simulink model "Receive1"  (R2021a)
settings: Solver=VariableStepAuto  StartTime=0.0  StopTime=20000  RelTol=1e-3
values from neighbouring files (symbols this model uses):
  n_overlapped_channel = 2 * 1024    (= 2048)    [receive1_script.m]
  parallel_factor = 4    [receive1_script.m]
libraries: xbsIndex_r4 x522, xrbsSSR_Library x15, dspsrcs4 x12
(part 1 of 4)
settings Model: Creator=11037  LastModifiedBy=11037

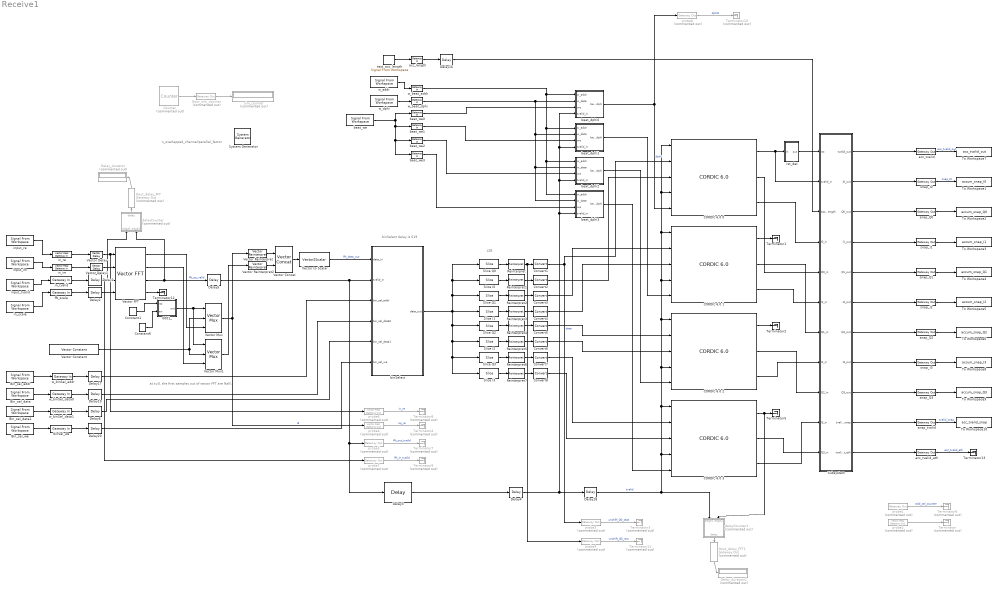
== system Receive1 ==
  note: binSelect delay is 519
  note: n_overlapped_channel/parallel_factor
  note: LSB
  note: at t=0, the first samples out of vector FFT are NaN,
  " System Generator" : xbsIndex_r4/ System Generator  Tag=genX  xilinxfamily=zynquplusRFSOC  part=xczu28dr  speed=-2-e  package=ffvg1517  synthesis_tool=Vivado  clock_wrapper=Clock Enables  directory=C:/Receive1_test_NL  proj_type=Vivado  Synth_file=Vivado Synthesis Defaults  Impl_file=Vivado Implementation Defaults  testbench=off  simulink_period=1  sysclk_period=10  dcm_input_clock_period=10  incr_netlist=off  trim_vbits=Everywhere in SubSystem  dbl_ovrd=According to Block Masks  core_generation=According to Block Masks  run_coregen=off  deprecated_control=off  eval_field=0  block_type=sysgen
  0001_ : Subsystem
  Bin_sel_addr : dspsrcs4/Signal From Workspace  X=15  Ts=1  nsamps=1  OutputAfterFinalValue=Holding final value  ignoreOrWarnInputAndFrameLengths=on  OutputFrames=off
  Bin_sel_data : dspsrcs4/Signal From Workspace  X=15  Ts=1  nsamps=1  OutputAfterFinalValue=Holding final value  ignoreOrWarnInputAndFrameLengths=on  OutputFrames=off
  Bin_sel_data1 : dspsrcs4/Signal From Workspace  X=15  Ts=1  nsamps=1  OutputAfterFinalValue=Holding final value  ignoreOrWarnInputAndFrameLengths=on  OutputFrames=off
  Bin_sel_we : dspsrcs4/Signal From Workspace  X=0  Ts=1  nsamps=1  OutputAfterFinalValue=Setting to zero  ignoreOrWarnInputAndFrameLengths=on  OutputFrames=off
  CORDIC 6.0 {0..3} (4 alike) : xbsIndex_r4/CORDIC 6.0   functional_selection=Rotate  architectural_configuration=Parallel  pipelining_mode=Optimal  data_format=SignedFraction  phase_format=Scaled_Radians  input_width=18  output_width=16  round_mode=Nearest_Even  iterations=16  precision=20  compensation_scaling=LUT_based  coarse_rotation=on  aclken=off  aresetn=off  out_tready=off  cartesian_has_tuser=off  cartesian_has_tlast=off  cartesian_tuser_width=1  phase_has_tuser=off  phase_has_tlast=off  phase_tuser_width=1  out_tlast_behv=Null  flow_control=NonBlocking  optimize_goal=Resources  trim_axipin_name=on  simulation_type=hybrid_sim  simulation_model=sysgen:cordic_v6_0  data_path_portlist={'s_axis_cartesian_tdata_imag', 's_axis_cartesian_tdata_real', 's_axis_phase_tdata_phase', 'm_axis_dout_tdata_imag', 'm_axis_dout_tdata_real', 'm_axis_dout_tdata_phase','m_axis_dout_tdata'}  ip_name=CORDIC  ip_version=6.0  dsptool_ready=true  ipcore_usecache=true  ipcore_useipmodelcache=true  wrapper_available=true  port_translation_map={ 'aclken' => 'en', 'aresetn' => 'rst' }  block_type=cordic_v6_0
      settings: infoedit=CORDIC 6.0
  Constant1 : xbsIndex_r4/Constant  const=0  gui_display_data_type=Boolean  arith_type=Boolean  n_bits=16  bin_pt=14  preci_type=Single  exp_width=8  frac_width=24  explicit_period=on  period=1  equ=P=C  opselect=C  inp2=PCIN>>17  opr=+  inp1=P  carry=CIN  dbl_ovrd=off  block_type=constant
  Constant6 : xbsIndex_r4/Constant  const=1  gui_display_data_type=Boolean  arith_type=Boolean  n_bits=16  bin_pt=14  preci_type=Single  exp_width=8  frac_width=24  explicit_period=on  period=1  equ=P=C  opselect=C  inp2=PCIN>>17  opr=+  inp1=P  carry=CIN  dbl_ovrd=off  block_type=constant
  Convert{1..8} (8 alike) : xbsIndex_r4/Convert  gui_display_data_type=Fixed-point  arith_type="Signed  (2's comp)"  n_bits=18  bin_pt=16  float_type=Single  exp_bits=8  fraction_bits=24  quantization=Truncate  overflow=Flag as error  en=off  latency=1  pipeline=off  dbl_ovrd=off  block_type=convert
  Counter : xbsIndex_r4/Counter  Commented=on  cnt_type=Free Running  cnt_to=Inf  operation=Up  start_count=0  cnt_by_val=1  arith_type=Unsigned  n_bits=24  bin_pt=0  load_pin=off  rst=off  en=off  explicit_period=on  period=1  use_behavioral_HDL=off  implementation=Fabric  dbl_ovrd=off  block_type=counter
  Delay1 : xbsIndex_r4/Delay  rst=off  infoeditControl=Selection of Reset will increase slice count due to use of real FFs and instead of SRLs  en=off  latency=1+15*256  reg_retiming=off  dbl_ovrd=off  block_type=delay
  Delay{2,4..6,16..17,19..20} (8 alike) : xbsIndex_r4/Delay  rst=off  infoeditControl=Selection of Reset will increase slice count due to use of real FFs and instead of SRLs  en=off  latency=1  reg_retiming=off  dbl_ovrd=off  block_type=delay
  Delay18 : xbsIndex_r4/Delay  rst=off  infoeditControl=Selection of Reset will increase slice count due to use of real FFs and instead of SRLs  en=off  latency=2  reg_retiming=off  dbl_ovrd=off  block_type=delay
  Delay3 : xbsIndex_r4/Delay  rst=off  infoeditControl=Selection of Reset will increase slice count due to use of real FFs and instead of SRLs  en=off  latency=519-2  reg_retiming=off  dbl_ovrd=off  block_type=delay
  Delay_duration : Display  Commented=on
  Delay_duration1 : Display  Commented=on
  Gout_delay_FFT : xbsIndex_r4/Gateway Out  Commented=on  inherit_from_input=on  hdl_port=on  rows=1  columns=1  UseAsDAC=off  DACChannel='1'  interface=None  automatic_assignment=on  address_offset=hex2dec('00')  intf_name=''  intf_description=''  timing_constraint=None  locs_specified=off  LOCs={}  io_standard={}  block_type=gatewayout
  Gout_delay_FFT1 : xbsIndex_r4/Gateway Out  Commented=on  inherit_from_input=on  hdl_port=on  rows=1  columns=1  UseAsDAC=off  DACChannel='1'  interface=None  automatic_assignment=on  address_offset=hex2dec('00')  intf_name=''  intf_description=''  timing_constraint=None  locs_specified=off  LOCs={}  io_standard={}  block_type=gatewayout
  Gout_sim_counter : xbsIndex_r4/Gateway Out  Commented=on  inherit_from_input=on  hdl_port=on  rows=1  columns=1  UseAsDAC=off  DACChannel='1'  interface=None  automatic_assignment=on  address_offset=hex2dec('00')  intf_name=''  intf_description=''  timing_constraint=None  locs_specified=off  LOCs={}  io_standard={}  block_type=gatewayout
  Reinterpret{,1..7} (8 alike) : xbsIndex_r4/Reinterpret  force_arith_type=on  arith_type="Signed  (2's comp)"  force_bin_pt=on  bin_pt=15  block_type=reinterpret
  Slice I0 : xbsIndex_r4/Slice  nbits=27  boolean_output=off  mode=Lower Bit Location + Width  bit1=0  base1=MSB of Input  bit0=27  base0=LSB of Input  dbl_ovrd=off  block_type=slice
  Slice I1 : xbsIndex_r4/Slice  nbits=27  boolean_output=off  mode=Lower Bit Location + Width  bit1=0  base1=MSB of Input  bit0=27*3  base0=LSB of Input  dbl_ovrd=off  block_type=slice
  Slice I2 : xbsIndex_r4/Slice  nbits=27  boolean_output=off  mode=Lower Bit Location + Width  bit1=0  base1=MSB of Input  bit0=27*5  base0=LSB of Input  dbl_ovrd=off  block_type=slice
  Slice I3 : xbsIndex_r4/Slice  nbits=27  boolean_output=off  mode=Lower Bit Location + Width  bit1=0  base1=MSB of Input  bit0=27*7  base0=LSB of Input  dbl_ovrd=off  block_type=slice
  Slice Q0 : xbsIndex_r4/Slice  nbits=27  boolean_output=off  mode=Lower Bit Location + Width  bit1=0  base1=MSB of Input  bit0=0  base0=LSB of Input  dbl_ovrd=off  block_type=slice
  Slice Q1 : xbsIndex_r4/Slice  nbits=27  boolean_output=off  mode=Lower Bit Location + Width  bit1=0  base1=MSB of Input  bit0=27*2  base0=LSB of Input  dbl_ovrd=off  block_type=slice
  Slice Q2 : xbsIndex_r4/Slice  nbits=27  boolean_output=off  mode=Lower Bit Location + Width  bit1=0  base1=MSB of Input  bit0=27*4  base0=LSB of Input  dbl_ovrd=off  block_type=slice
  Slice Q3 : xbsIndex_r4/Slice  nbits=27  boolean_output=off  mode=Lower Bit Location + Width  bit1=0  base1=MSB of Input  bit0=27*6  base0=LSB of Input  dbl_ovrd=off  block_type=slice
  Subsystem : Subsystem
  Terminator{,3..4,6..11} (9 alike) : Terminator  Commented=on
  Terminator{1..2,5,12..13} (5 alike) : Terminator
  To Workspace1 : ToWorkspace  VariableName=accum_snap_I0  SampleTime=1
  To Workspace10 : ToWorkspace  VariableName=acc_tvalid_snap  SampleTime=1
  To Workspace2 : ToWorkspace  VariableName=accum_snap_Q0  SampleTime=1
  To Workspace3 : ToWorkspace  VariableName=accum_snap_I1  SampleTime=1
  To Workspace4 : ToWorkspace  VariableName=accum_snap_Q1  SampleTime=1
  To Workspace5 : ToWorkspace  VariableName=accum_snap_I2  SampleTime=1
  To Workspace6 : ToWorkspace  VariableName=accum_snap_Q2  SampleTime=1
  To Workspace7 : ToWorkspace  VariableName=acc_tvalid_out  SampleTime=1
  To Workspace8 : ToWorkspace  VariableName=accum_snap_I3  SampleTime=1
  To Workspace9 : ToWorkspace  VariableName=accum_snap_Q3  SampleTime=1
  Vector Concat : xrbsSSR_Library/Vector Concat  num_inputs=2  num_inputs_prev=2  sg_ssr=4  sg_ssr_prev=4  dbl_ovrd=off  block_type=concat_ssr  sg_ssr_name=vect_concat
      settings: SourceProductName=Xilinx SSR Blockset  infoedit=The Vector Concat block concatenates two or more inputs of type vector. Output will be cast to an unsigned value with the binary point at zero.
  Vector Constant : xrbsSSR_Library/Vector Constant  const=[0.9 0.9 0.9 0.9]  gui_display_data_type=Fixed-point  arith_type=Signed (2's comp)  n_bits=16  bin_pt=15  preci_type=Single  exp_width=8  frac_width=24  explicit_period=on  period=1  sg_ssr=4  sg_ssr_prev=4  equ=P=C  opselect=C  inp2=PCIN>>17  opr=+  inp1=P  carry=CIN  dbl_ovrd=off  block_type=constant_ssr
      settings: SourceProductName=Xilinx SSR Blockset
  Vector Delay : xrbsSSR_Library/Vector Delay  sg_latency=1  infoeditControl=Selection of Reset will increase slice count due to use of real FFs and instead of SRLs  en=off  vectorize_en=off  rst=off  reg_retiming=off  block_type=delay_ssr  dbl_ovrd=off  sg_ssr=4  sg_ssr_prev=4  sg_ssr_name=vect_delay
      settings: SourceProductName=Xilinx SSR Blockset
  Vector Delay1 : xrbsSSR_Library/Vector Delay  sg_latency=1  infoeditControl=Selection of Reset will increase slice count due to use of real FFs and instead of SRLs  en=off  vectorize_en=off  rst=off  reg_retiming=off  block_type=delay_ssr  dbl_ovrd=off  sg_ssr=4  sg_ssr_prev=4  sg_ssr_name=vect_delay
      settings: SourceProductName=Xilinx SSR Blockset
  Vector FFT : xrbsSSR_Library/Vector FFT  sg_ssr=4  N=2048  W_high=1  W_low=-17  n_bits=27  bin_pt=14+1  bram_threshold=258  block_type=fft_ssr  sg_ssr_prev=4
      settings: SourceProductName=Xilinx SSR Blockset
  Vector Mux : xrbsSSR_Library/Vector Mux  inputs=2  inputs_prev=2  en=off  vectorize_en=off  vectorize_sel=off  sg_latency=1  precision=User Defined  arith_type="Signed  (2's comp)"  n_bits=27  bin_pt=15  quantization=Truncate  overflow=Saturate  dbl_ovrd=off  block_type=mux_ssr  sg_ssr=4  sg_ssr_prev=4  sg_ssr_name=vect_mux
      settings: SourceProductName=Xilinx SSR Blockset  infoedit=The Vector Multiplexer block supports Multiplexing feature for input of vector types.
  Vector Mux1 : xrbsSSR_Library/Vector Mux  inputs=2  inputs_prev=2  en=off  vectorize_en=off  vectorize_sel=off  sg_latency=1  precision=User Defined  arith_type="Signed  (2's comp)"  n_bits=27  bin_pt=15  quantization=Truncate  overflow=Saturate  dbl_ovrd=off  block_type=mux_ssr  sg_ssr=4  sg_ssr_prev=4  sg_ssr_name=vect_mux
      settings: SourceProductName=Xilinx SSR Blockset  infoedit=The Vector Multiplexer block supports Multiplexing feature for input of vector types.
  Vector Reinterpret : xrbsSSR_Library/Vector Reinterpret  sg_ssr=4  sg_ssr_prev=4  force_arith_type=on  arith_type=Unsigned  force_bin_pt=on  bin_pt=0  block_type=reinterpret_ssr
      settings: SourceProductName=Xilinx SSR Blockset  infoedit="The Vector Reinterpret block Changes vector input signal type without altering the binary representation. You can change the signal between signed and unsigned, and relocate the binary point.<br><br>Hardware notes: In hardware this block costs nothing.<br><br>Example:  Suppose the input is 6 bits wide, signed, with 2 fractional bits, and the output is forced to unsigned with 0 fractional bits.  Then an input of -2.0 (1110.00 in binary 2's complement) becomes an output of 56 (111000 in binary)."
  Vector Reinterpret2 : xrbsSSR_Library/Vector Reinterpret  sg_ssr=4  sg_ssr_prev=4  force_arith_type=on  arith_type=Unsigned  force_bin_pt=on  bin_pt=0  block_type=reinterpret_ssr
      settings: SourceProductName=Xilinx SSR Blockset  infoedit="The Vector Reinterpret block Changes vector input signal type without altering the binary representation. You can change the signal between signed and unsigned, and relocate the binary point.<br><br>Hardware notes: In hardware this block costs nothing.<br><br>Example:  Suppose the input is 6 bits wide, signed, with 2 fractional bits, and the output is forced to unsigned with 0 fractional bits.  Then an input of -2.0 (1110.00 in binary 2's complement) becomes an output of 56 (111000 in binary)."
  Vector to Scalar : xrbsSSR_Library/Vector2Scalar  sg_ssr=4  sg_ssr_prev=4  sg_ssr_name=vect_Vector2Scalar  block_type=vector2scalar_ssr
      settings: SourceProductName=Xilinx SSR Blockset
  acc_length : xbsIndex_r4/Gateway In  gui_display_data_type=Fixed-point  arith_type=Unsigned  n_bits=23  bin_pt=0  preci_type=Single  exp_width=8  frac_width=24  rows=1  columns=1  quantization=Truncate  overflow=Flag as error  period=1  UseAsADC=off  ADCChannel='1'  interface=None  automatic_assignment=on  address_offset=hex2dec('00')  intf_name=''  intf_description=''  default_value=0  timing_constraint=None  locs_specified=off  LOCs={}  io_standard={}  inherit_from_input=off  hdl_port=on  dbl_ovrd=off  block_type=gatewayin
  acc_tvalid : xbsIndex_r4/Gateway Out  inherit_from_input=off  hdl_port=on  rows=1  columns=1  UseAsDAC=off  DACChannel='1'  interface=None  automatic_assignment=on  address_offset=hex2dec('00')  intf_name=''  intf_description=''  timing_constraint=None  locs_specified=off  LOCs={}  io_standard={}  block_type=gatewayout
  acc_tvalid_eth : xbsIndex_r4/Gateway Out  inherit_from_input=off  hdl_port=on  rows=1  columns=1  UseAsDAC=off  DACChannel='1'  interface=None  automatic_assignment=on  address_offset=hex2dec('00')  intf_name=''  intf_description=''  timing_constraint=None  locs_specified=off  LOCs={}  io_standard={}  block_type=gatewayout
  beat_dphi0 : Subsystem
  beat_dphi1 : Subsystem
  beat_dphi2 : Subsystem
  beat_dphi3 : Subsystem
  beat_we : dspsrcs4/Signal From Workspace  X=0  Ts=1  nsamps=1  OutputAfterFinalValue=Holding final value  ignoreOrWarnInputAndFrameLengths=on  OutputFrames=off
  beat_we{0..3} (4 alike) : xbsIndex_r4/Gateway In  gui_display_data_type=Boolean  arith_type=Boolean  n_bits=16  bin_pt=0  preci_type=Single  exp_width=8  frac_width=24  rows=1  columns=1  quantization=Truncate  overflow=Flag as error  period=1  UseAsADC=off  ADCChannel='1'  interface=None  automatic_assignment=on  address_offset=hex2dec('00')  intf_name=''  intf_description=''  default_value=0  timing_constraint=None  locs_specified=off  LOCs={}  io_standard={}  inherit_from_input=off  hdl_port=on  dbl_ovrd=off  block_type=gatewayin
  binSel_we : xbsIndex_r4/Gateway In  gui_display_data_type=Boolean  arith_type=Boolean  n_bits=16  bin_pt=14  preci_type=Single  exp_width=8  frac_width=24  rows=1  columns=1  quantization="Round  (unbiased: +/- Inf)"  overflow=Saturate  period=1  UseAsADC=off  ADCChannel='1'  interface=None  automatic_assignment=on  address_offset=hex2dec('00')  intf_name=''  intf_description=''  default_value=0  timing_constraint=None  locs_specified=off  LOCs={}  io_standard={}  inherit_from_input=off  hdl_port=on  dbl_ovrd=off  block_type=gatewayin
  binSelect : Subsystem
  delayCounter : Subsystem  Commented=on
  delayCounter1 : Subsystem  Commented=on
  fft_scale : xbsIndex_r4/Gateway In  gui_display_data_type=Fixed-point  arith_type=Unsigned  n_bits=11  bin_pt=0  preci_type=Single  exp_width=8  frac_width=24  rows=1  columns=1  quantization=Truncate  overflow=Wrap  period=1  UseAsADC=off  ADCChannel='1'  interface=None  automatic_assignment=on  address_offset=hex2dec('00')  intf_name=''  intf_description=''  default_value=0  timing_constraint=None  locs_specified=off  LOCs={}  io_standard={}  inherit_from_input=off  hdl_port=on  dbl_ovrd=off  block_type=gatewayin
  in_im : xrbsSSR_Library/Vector Real Gateway In  gui_display_data_type=Fixed-point  arith_type="Signed  (2's comp)"  n_bits=16  bin_pt=14  preci_type=Single  exp_width=8  frac_width=24  quantization=Truncate  overflow=Wrap  period=1  sg_ssr=4  sg_ssr_prev=4  UseAsADC=off  ADCChannel='1'  interface=None  interface_prev=1  automatic_assignment=off  address_offset=hex2dec('00')  intf_name=''  intf_description=''  default_value=0  timing_constraint=None  locs_specified=off  LOCs={}  io_standard={}  hdl_port=on  dbl_ovrd=off  block_type=realgatewayin_ssr
      settings: SourceProductName=Xilinx SSR Blockset  infoedit=The Vector Real Gateway in block converts Vector inputs of type Simulink integer, single, double and fixed-point to Xilinx fixed-point or floating-point data type.<br><br>Hardware notes: In hardware these blocks become top level input ports.
  in_re : xrbsSSR_Library/Vector Real Gateway In  gui_display_data_type=Fixed-point  arith_type="Signed  (2's comp)"  n_bits=16  bin_pt=14  preci_type=Single  exp_width=8  frac_width=24  quantization=Truncate  overflow=Wrap  period=1  sg_ssr=4  sg_ssr_prev=4  UseAsADC=off  ADCChannel='1'  interface=None  interface_prev=1  automatic_assignment=off  address_offset=hex2dec('00')  intf_name=''  intf_description=''  default_value=0  timing_constraint=None  locs_specified=off  LOCs={}  io_standard={}  hdl_port=on  dbl_ovrd=off  block_type=realgatewayin_ssr
      settings: SourceProductName=Xilinx SSR Blockset  infoedit=The Vector Real Gateway in block converts Vector inputs of type Simulink integer, single, double and fixed-point to Xilinx fixed-point or floating-point data type.<br><br>Hardware notes: In hardware these blocks become top level input ports.
  in_scale : dspsrcs4/Signal From Workspace  X=2016  Ts=1  nsamps=1  OutputAfterFinalValue=Holding final value  ignoreOrWarnInputAndFrameLengths=on  OutputFrames=off
  in_tvalid : xbsIndex_r4/Gateway In  gui_display_data_type=Boolean  arith_type=Boolean  n_bits=16  bin_pt=14  preci_type=Single  exp_width=8  frac_width=24  rows=1  columns=1  quantization="Round  (unbiased: +/- Inf)"  overflow=Saturate  period=1  UseAsADC=off  ADCChannel='1'  interface=None  automatic_assignment=on  address_offset=hex2dec('00')  intf_name=''  intf_description=''  default_value=0  timing_constraint=None  locs_specified=off  LOCs={}  io_standard={}  inherit_from_input=off  hdl_port=on  dbl_ovrd=off  block_type=gatewayin
  input_im : dspsrcs4/Signal From Workspace  X=PSB_out_im  Ts=1  nsamps=1  OutputAfterFinalValue=Setting to zero  ignoreOrWarnInputAndFrameLengths=on  OutputFrames=off
  input_re : dspsrcs4/Signal From Workspace  X=PSB_out_re  Ts=1  nsamps=1  OutputAfterFinalValue=Setting to zero  ignoreOrWarnInputAndFrameLengths=on  OutputFrames=off
  input_tvalid : dspsrcs4/Signal From Workspace  X=PSB_out_tvalid  Ts=1  nsamps=1  OutputAfterFinalValue=Setting to zero  ignoreOrWarnInputAndFrameLengths=on  OutputFrames=off
  probe{1,3,5,7..9} (6 alike) : xbsIndex_r4/Gateway Out  Commented=on  inherit_from_input=off  hdl_port=on  rows=1  columns=1  UseAsDAC=off  DACChannel='1'  interface=None  automatic_assignment=on  address_offset=hex2dec('00')  intf_name=''  intf_description=''  timing_constraint=None  locs_specified=off  LOCs={}  io_standard={}  block_type=gatewayout
  probe2 : xrbsSSR_Library/Vector Real Gateway Out  Commented=on  inherit_from_input=off  hdl_port=on  rows=1  columns=1  UseAsDAC=off  DACChannel='1'  interface=None  automatic_assignment=on  address_offset=hex2dec('00')  intf_name=''  intf_description=''  timing_constraint=None  locs_specified=off  LOCs={}  io_standard={}  block_type=realgatewayout_ssr  sg_ssr=4  sg_ssr_prev=4  sg_ssr_name=vect_real_gwayout
      settings: SourceProductName=Xilinx SSR Blockset  infoedit=The Vector Real Gateway out block converts Xilinx fixed-point or floating-point type vector inputs into vector ouputs of type Simulink integer, single, double, or fixed-point.<br><br>Hardware notes: In hardware these blocks become top level output ports or are discarded, depending on how they are configured.
  probe4 : xrbsSSR_Library/Vector Real Gateway Out  Commented=on  inherit_from_input=off  hdl_port=on  rows=1  columns=1  UseAsDAC=off  DACChannel='1'  interface=None  automatic_assignment=on  address_offset=hex2dec('00')  intf_name=''  intf_description=''  timing_constraint=None  locs_specified=off  LOCs={}  io_standard={}  block_type=realgatewayout_ssr  sg_ssr=4  sg_ssr_prev=4  sg_ssr_name=vect_real_gwayout
      settings: SourceProductName=Xilinx SSR Blockset  infoedit=The Vector Real Gateway out block converts Xilinx fixed-point or floating-point type vector inputs into vector ouputs of type Simulink integer, single, double, or fixed-point.<br><br>Hardware notes: In hardware these blocks become top level output ports or are discarded, depending on how they are configured.
  probe6 : xrbsSSR_Library/Vector Real Gateway Out  Commented=on  inherit_from_input=off  hdl_port=on  rows=1  columns=1  UseAsDAC=off  DACChannel='1'  interface=None  automatic_assignment=on  address_offset=hex2dec('00')  intf_name=''  intf_description=''  timing_constraint=None  locs_specified=off  LOCs={}  io_standard={}  block_type=realgatewayout_ssr  sg_ssr=4  sg_ssr_prev=4  sg_ssr_name=vect_real_gwayout
      settings: SourceProductName=Xilinx SSR Blockset  infoedit=The Vector Real Gateway out block converts Xilinx fixed-point or floating-point type vector inputs into vector ouputs of type Simulink integer, single, double, or fixed-point.<br><br>Hardware notes: In hardware these blocks become top level output ports or are discarded, depending on how they are configured.
  rst_det : Subsystem
  sim_counter : Display  Commented=on
      settings: Format=decimal (Stored Integer)
  snap_I{0..3} (4 alike) : xbsIndex_r4/Gateway Out  inherit_from_input=off  hdl_port=on  rows=1  columns=1  UseAsDAC=off  DACChannel='1'  interface=None  automatic_assignment=on  address_offset=hex2dec('00')  intf_name=''  intf_description=''  timing_constraint=None  locs_specified=off  LOCs={}  io_standard={}  block_type=gatewayout
  snap_Q{0..3} (4 alike) : xbsIndex_r4/Gateway Out  inherit_from_input=off  hdl_port=on  rows=1  columns=1  UseAsDAC=off  DACChannel='1'  interface=None  automatic_assignment=on  address_offset=hex2dec('00')  intf_name=''  intf_description=''  timing_constraint=None  locs_specified=off  LOCs={}  io_standard={}  block_type=gatewayout
  snap_tvalid : xbsIndex_r4/Gateway Out  inherit_from_input=off  hdl_port=on  rows=1  columns=1  UseAsDAC=off  DACChannel='1'  interface=None  automatic_assignment=on  address_offset=hex2dec('00')  intf_name=''  intf_description=''  timing_constraint=None  locs_specified=off  LOCs={}  io_standard={}  block_type=gatewayout
  test_acc_length : dspsrcs4/Signal From Workspace  X=acc_length  Ts=1  nsamps=1  OutputAfterFinalValue=Holding final value  ignoreOrWarnInputAndFrameLengths=on  OutputFrames=off
  w_addr : dspsrcs4/Signal From Workspace  X=[0:511]  Ts=1  nsamps=1  OutputAfterFinalValue=Cyclic repetition  ignoreOrWarnInputAndFrameLengths=on  OutputFrames=off
  w_beat_addr : xbsIndex_r4/Gateway In  gui_display_data_type=Fixed-point  arith_type=Unsigned  n_bits=9  bin_pt=0  preci_type=Single  exp_width=8  frac_width=24  rows=1  columns=1  quantization=Truncate  overflow=Flag as error  period=1  UseAsADC=off  ADCChannel='1'  interface=None  automatic_assignment=on  address_offset=hex2dec('00')  intf_name=''  intf_description=''  default_value=0  timing_constraint=None  locs_specified=off  LOCs={}  io_standard={}  inherit_from_input=off  hdl_port=on  dbl_ovrd=off  block_type=gatewayin
  w_beat_dphi : xbsIndex_r4/Gateway In  gui_display_data_type=Fixed-point  arith_type=Unsigned  n_bits=16  bin_pt=0  preci_type=Single  exp_width=8  frac_width=24  rows=1  columns=1  quantization=Truncate  overflow=Flag as error  period=1  UseAsADC=off  ADCChannel='1'  interface=None  automatic_assignment=on  address_offset=hex2dec('00')  intf_name=''  intf_description=''  default_value=0  timing_constraint=None  locs_specified=off  LOCs={}  io_standard={}  inherit_from_input=off  hdl_port=on  dbl_ovrd=off  block_type=gatewayin
  w_binSel_addr : xbsIndex_r4/Gateway In  gui_display_data_type=Fixed-point  arith_type=Unsigned  n_bits=10  bin_pt=0  preci_type=Single  exp_width=8  frac_width=24  rows=1  columns=1  quantization=Truncate  overflow=Flag as error  period=1  UseAsADC=off  ADCChannel='1'  interface=None  automatic_assignment=on  address_offset=hex2dec('00')  intf_name=''  intf_description=''  default_value=0  timing_constraint=None  locs_specified=off  LOCs={}  io_standard={}  inherit_from_input=off  hdl_port=on  dbl_ovrd=off  block_type=gatewayin
  w_binSel_data0 : xbsIndex_r4/Gateway In  gui_display_data_type=Fixed-point  arith_type=Unsigned  n_bits=22  bin_pt=0  preci_type=Single  exp_width=8  frac_width=24  rows=1  columns=1  quantization=Truncate  overflow=Flag as error  period=1  UseAsADC=off  ADCChannel='1'  interface=None  automatic_assignment=on  address_offset=hex2dec('00')  intf_name=''  intf_description=''  default_value=0  timing_constraint=None  locs_specified=off  LOCs={}  io_standard={}  inherit_from_input=off  hdl_port=on  dbl_ovrd=off  block_type=gatewayin
  w_binSel_data1 : xbsIndex_r4/Gateway In  gui_display_data_type=Fixed-point  arith_type=Unsigned  n_bits=22  bin_pt=0  preci_type=Single  exp_width=8  frac_width=24  rows=1  columns=1  quantization=Truncate  overflow=Flag as error  period=1  UseAsADC=off  ADCChannel='1'  interface=None  automatic_assignment=on  address_offset=hex2dec('00')  intf_name=''  intf_description=''  default_value=0  timing_constraint=None  locs_specified=off  LOCs={}  io_standard={}  inherit_from_input=off  hdl_port=on  dbl_ovrd=off  block_type=gatewayin
  w_dphi : dspsrcs4/Signal From Workspace  X=beat_dphi_uint16_0  Ts=1  nsamps=1  OutputAfterFinalValue=Cyclic repetition  ignoreOrWarnInputAndFrameLengths=on  OutputFrames=off
  wires:
  Vector Concat/1 -> Vector to Scalar/1
  Vector FFT/3 -> Delay5/1, delayCounter/2(edge2)  "fft_op_valid"
  input_re/1 -> in_re/1
  Vector FFT/4 -> Terminator12/1
  input_tvalid/1 -> in_tvalid/1
  input_im/1 -> in_im/1
  in_scale/1 -> fft_scale/1
  in_re/1 -> Vector Delay/1
  Vector Delay/1 -> probe6/1, Vector FFT/1
  in_im/1 -> Vector Delay1/1
  Vector Delay1/1 -> Vector FFT/2
  in_tvalid/1 -> Delay1/1
  Delay1/1 -> probe7/1, Vector FFT/3, delayCounter/1(edge1)
  fft_scale/1 -> Delay2/1
  Delay2/1 -> Vector FFT/4
  Vector Reinterpret/1 -> Vector Concat/1
  Vector Reinterpret2/1 -> Vector Concat/2
  Slice Q0/1 -> Reinterpret/1
  Slice I1/1 -> Reinterpret3/1
  Slice Q1/1 -> Reinterpret2/1
  Slice I2/1 -> Reinterpret5/1
  Slice Q2/1 -> Reinterpret4/1
  Slice I3/1 -> Reinterpret7/1
  Slice Q3/1 -> Reinterpret6/1
  Slice I0/1 -> Reinterpret1/1
  Delay3/1 -> Delay4/1
  w_dphi/1 -> w_beat_dphi/1
  w_addr/1 -> w_beat_addr/1
  acc_tvalid/1 -> To Workspace7/1  "acc_tvalid_out"
  snap_I0/1 -> To Workspace1/1  "snap_I0"
  test_acc_length/1 -> acc_length/1
  acc_length/1 -> Delay16/1
  CORDIC 6.0 0/1 -> rst_det/1(in), Subsystem/2(tvalid_in)
  CORDIC 6.0 1/1 -> Terminator1/1
  CORDIC 6.0 0/3 -> Subsystem/4(I0_in)
  CORDIC 6.0 0/2 -> Subsystem/5(Q0_in)
  CORDIC 6.0 1/3 -> Subsystem/6(I1_in)
  CORDIC 6.0 1/2 -> Subsystem/7(Q1_in)
  CORDIC 6.0 2/3 -> Subsystem/8(I2_in)
  CORDIC 6.0 2/2 -> Subsystem/9(Q2_in)
  CORDIC 6.0 3/3 -> Subsystem/10(I3_in)
  CORDIC 6.0 3/2 -> Subsystem/11(Q3_in)
  CORDIC 6.0 2/1 -> Terminator2/1
  CORDIC 6.0 3/1 -> delayCounter1/2(edge2), Terminator5/1
  Subsystem/1(tvalid_out) -> acc_tvalid/1
  Subsystem/2(I0_out) -> snap_I0/1
  snap_Q0/1 -> To Workspace2/1
  Subsystem/3(Q0_out) -> snap_Q0/1
  snap_Q1/1 -> To Workspace4/1
  snap_I1/1 -> To Workspace3/1
  snap_Q2/1 -> To Workspace6/1
  snap_I2/1 -> To Workspace5/1
  snap_Q3/1 -> To Workspace9/1
  snap_I3/1 -> To Workspace8/1
  Subsystem/9(Q3_out) -> snap_Q3/1
  Subsystem/8(I3_out) -> snap_I3/1
  Subsystem/7(Q2_out) -> snap_Q2/1
  Subsystem/6(I2_out) -> snap_I2/1
  Subsystem/5(Q1_out) -> snap_Q1/1
  Subsystem/4(I1_out) -> snap_I1/1
  beat_we/1 -> beat_we0/1, beat_we1/1, beat_we2/1, beat_we3/1
  Delay18/1 -> delayCounter1/1(edge1), CORDIC 6.0 3/1, CORDIC 6.0 0/4, CORDIC 6.0 0/1, CORDIC 6.0 1/1, CORDIC 6.0 1/4, CORDIC 6.0 2/1, CORDIC 6.0 2/4, CORDIC 6.0 3/4  "tvalid"
  w_beat_addr/1 -> beat_dphi0/1(w_addr), beat_dphi1/1(w_addr), beat_dphi3/1(w_addr), beat_dphi2/1(w_addr)
  w_beat_dphi/1 -> beat_dphi0/2(w_data), beat_dphi1/2(w_data), beat_dphi3/2(w_data), beat_dphi2/2(w_data)
  beat_we0/1 -> beat_dphi0/3(we)
  beat_dphi0/1(beat_dphi) -> probe8/1, CORDIC 6.0 0/5  "dphi"
  beat_dphi1/1(beat_dphi) -> CORDIC 6.0 1/5
  beat_dphi2/1(beat_dphi) -> CORDIC 6.0 2/5
  beat_dphi3/1(beat_dphi) -> CORDIC 6.0 3/5
  beat_we1/1 -> beat_dphi1/3(we)
  beat_we2/1 -> beat_dphi2/3(we)
  beat_we3/1 -> beat_dphi3/3(we)
  Delay16/1 -> Subsystem/3(acc_length)
  Reinterpret/1 -> probe9/1, Convert1/1
  Reinterpret1/1 -> Convert2/1
  Reinterpret2/1 -> Convert3/1
  Reinterpret3/1 -> Convert4/1
  Reinterpret4/1 -> Convert5/1
  Reinterpret5/1 -> Convert6/1
  Reinterpret6/1 -> Convert7/1
  Reinterpret7/1 -> Convert8/1
  Convert1/1 -> probe3/1, CORDIC 6.0 0/2  "data"
  Convert2/1 -> CORDIC 6.0 0/3
  Convert3/1 -> CORDIC 6.0 1/2
  Convert4/1 -> CORDIC 6.0 1/3
  Convert5/1 -> CORDIC 6.0 2/2
  Convert6/1 -> CORDIC 6.0 2/3
  Convert7/1 -> CORDIC 6.0 3/2
  Convert8/1 -> CORDIC 6.0 3/3
  w_binSel_addr/1 -> Delay17/1
  w_binSel_data0/1 -> Delay19/1
  binSel_we/1 -> Delay20/1
  Bin_sel_addr/1 -> w_binSel_addr/1
  Bin_sel_data/1 -> w_binSel_data0/1
  Bin_sel_we/1 -> binSel_we/1
  binSelect/1(data_out) -> Slice I3/1, Slice Q3/1, Slice I2/1, Slice Q2/1, Slice I0/1, Slice Q0/1, Slice Q1/1, Slice I1/1
  Vector to Scalar/1 -> binSelect/1(data_in)  "fft_data_out"
  Delay17/1 -> binSelect/3(bin_sel_addr)
  Delay19/1 -> binSelect/4(bin_sel_data0)
  Delay20/1 -> binSelect/6(bin_sel_we)
  Delay4/1 -> Delay18/1, beat_dphi3/4(tvalid_in), beat_dphi2/4(tvalid_in), beat_dphi1/4(tvalid_in), beat_dphi0/4(tvalid_in)
  Gout_delay_FFT/1 -> Delay_duration/1
  delayCounter/1(delay) -> Gout_delay_FFT/1
  rst_det/1(out) -> Subsystem/1(rst)
  delayCounter1/1(delay) -> Gout_delay_FFT1/1
  Gout_delay_FFT1/1 -> Delay_duration1/1
  snap_tvalid/1 -> To Workspace10/1  "tvalid_snap"
  Subsystem/10(tvalid_snap) -> snap_tvalid/1
  probe1/1 -> Terminator6/1  "add_sel_counter"
  probe2/1 -> Terminator/1
  probe3/1 -> Terminator3/1  "unshift_Q0_cast"
  probe4/1 -> Terminator4/1  "op_re"
  probe5/1 -> Terminator7/1  "fft_out_tvalid"
  probe6/1 -> Terminator8/1  "in_re"
  probe7/1 -> Terminator9/1  "fft_in_tvalid"
  Counter/1 -> Gout_sim_counter/1
  Gout_sim_counter/1 -> sim_counter/1
  probe8/1 -> Terminator10/1  "dphi0"
  probe9/1 -> Terminator11/1  "unshift_Q0_raw"
  Vector Constant/1 -> Vector Mux/2, Vector Mux1/2
  0001_/1(out) -> Vector Mux1/1, Vector Mux/1
  Constant6/1 -> 0001_/2(en)
  Constant1/1 -> 0001_/1(rst)
  Delay5/1 -> Delay3/1, probe5/1, binSelect/2(tvalid_in)
  Vector FFT/1 -> Vector Mux/3
  Vector FFT/2 -> Vector Mux1/3
  Vector Mux/1 -> Vector Reinterpret/1, probe4/1  "B"
  Vector Mux1/1 -> Vector Reinterpret2/1
  w_binSel_data1/1 -> Delay6/1
  Bin_sel_data1/1 -> w_binSel_data1/1
  Delay6/1 -> binSelect/5(bin_sel_data1)
  Subsystem/11(tvalid_out_eth) -> acc_tvalid_eth/1
  acc_tvalid_eth/1 -> Terminator13/1  "acc_tvalid_eth"

== system Receive1/0001_ ==
  rst : Inport
  en : Inport  Port=2
  Constant17 : xbsIndex_r4/Constant  const=3  gui_display_data_type=Fixed-point  arith_type=Unsigned  n_bits=2  bin_pt=0  preci_type=Single  exp_width=8  frac_width=24  explicit_period=on  period=1  equ=P=C  opselect=C  inp2=PCIN>>17  opr=+  inp1=P  carry=CIN  dbl_ovrd=off  block_type=constant
  Counter : xbsIndex_r4/Counter  cnt_type=Free Running  cnt_to=3  operation=Up  start_count=0  cnt_by_val=1  arith_type=Unsigned  n_bits=2  bin_pt=0  load_pin=off  rst=on  en=on  explicit_period=on  period=1  use_behavioral_HDL=off  implementation=Fabric  dbl_ovrd=off  block_type=counter
  Register : xbsIndex_r4/Register  init=0  rst=on  en=on  dbl_ovrd=off  block_type=register
  Relational : xbsIndex_r4/Relational  mode=a>=b  op_type=Bool  en=off  latency=1  dbl_ovrd=off  block_type=relational
  const : xbsIndex_r4/Constant  const=1  gui_display_data_type=Boolean  arith_type=Boolean  n_bits=18  bin_pt=16  preci_type=Single  exp_width=8  frac_width=24  explicit_period=on  period=1  equ=P=C  opselect=C  inp2=PCIN>>17  opr=+  inp1=P  carry=CIN  dbl_ovrd=off  block_type=constant
  out : Outport
  wires:
  Counter/1 -> Relational/1
  const/1 -> Register/1
  rst/1 -> Counter/1, Register/2
  Register/1 -> out/1
  Constant17/1 -> Relational/2
  Relational/1 -> Register/3
  en/1 -> Counter/2

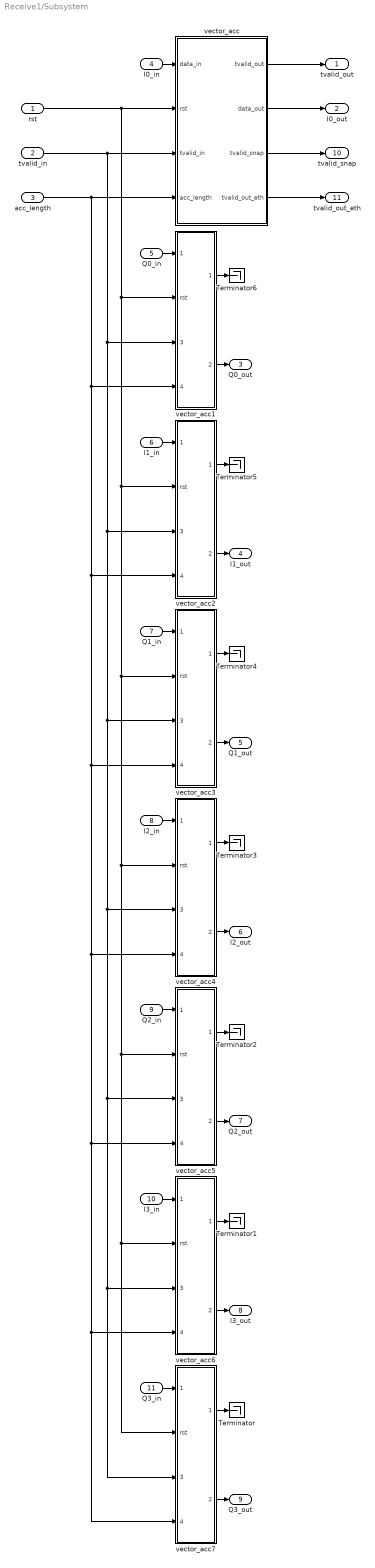
== system Receive1/Subsystem ==
  rst : Inport
  tvalid_in : Inport  Port=2
  acc_length : Inport  Port=3
  I0_in : Inport  Port=4
  Q0_in : Inport  Port=5
  I1_in : Inport  Port=6
  Q1_in : Inport  Port=7
  I2_in : Inport  Port=8
  Q2_in : Inport  Port=9
  I3_in : Inport  Port=10
  Q3_in : Inport  Port=11
  Terminator{,1..6} (7 alike) : Terminator
  vector_acc : Subsystem
  vector_acc1 : Subsystem
  vector_acc2 : Subsystem
  vector_acc3 : Subsystem
  vector_acc4 : Subsystem
  vector_acc5 : Subsystem
  vector_acc6 : Subsystem
  vector_acc7 : Subsystem
  tvalid_out : Outport
  I0_out : Outport  Port=2
  Q0_out : Outport  Port=3
  I1_out : Outport  Port=4
  Q1_out : Outport  Port=5
  I2_out : Outport  Port=6
  Q2_out : Outport  Port=7
  I3_out : Outport  Port=8
  Q3_out : Outport  Port=9
  tvalid_snap : Outport  Port=10
  tvalid_out_eth : Outport  Port=11
  wires:
  rst/1 -> vector_acc1/2(rst), vector_acc2/2(rst), vector_acc3/2(rst), vector_acc4/2(rst), vector_acc5/2(rst), vector_acc7/2(rst), vector_acc6/2(rst), vector_acc/2(rst)
  acc_length/1 -> vector_acc1/4(acc_length), vector_acc2/4(acc_length), vector_acc3/4(acc_length), vector_acc4/4(acc_length), vector_acc5/4(acc_length), vector_acc7/4(acc_length), vector_acc6/4(acc_length), vector_acc/4(acc_length)
  vector_acc7/2(data_out) -> Q3_out/1
  Q2_in/1 -> vector_acc5/1(data_in)
  Q3_in/1 -> vector_acc7/1(data_in)
  vector_acc3/2(data_out) -> Q1_out/1
  I2_in/1 -> vector_acc4/1(data_in)
  vector_acc7/1(tvalid_out) -> Terminator/1
  vector_acc6/1(tvalid_out) -> Terminator1/1
  tvalid_in/1 -> vector_acc1/3(tvalid_in), vector_acc2/3(tvalid_in), vector_acc3/3(tvalid_in), vector_acc4/3(tvalid_in), vector_acc5/3(tvalid_in), vector_acc7/3(tvalid_in), vector_acc6/3(tvalid_in), vector_acc/3(tvalid_in)
  I1_in/1 -> vector_acc2/1(data_in)
  vector_acc/1(tvalid_out) -> tvalid_out/1
  I3_in/1 -> vector_acc6/1(data_in)
  vector_acc6/2(data_out) -> I3_out/1
  vector_acc4/1(tvalid_out) -> Terminator3/1
  vector_acc3/1(tvalid_out) -> Terminator4/1
  vector_acc2/2(data_out) -> I1_out/1
  vector_acc4/2(data_out) -> I2_out/1
  I0_in/1 -> vector_acc/1(data_in)
  vector_acc/2(data_out) -> I0_out/1
  Q1_in/1 -> vector_acc3/1(data_in)
  vector_acc5/2(data_out) -> Q2_out/1
  vector_acc5/1(tvalid_out) -> Terminator2/1
  vector_acc2/1(tvalid_out) -> Terminator5/1
  vector_acc1/2(data_out) -> Q0_out/1
  vector_acc1/1(tvalid_out) -> Terminator6/1
  Q0_in/1 -> vector_acc1/1(data_in)
  vector_acc/3(tvalid_snap) -> tvalid_snap/1
  vector_acc/4(tvalid_out_eth) -> tvalid_out_eth/1

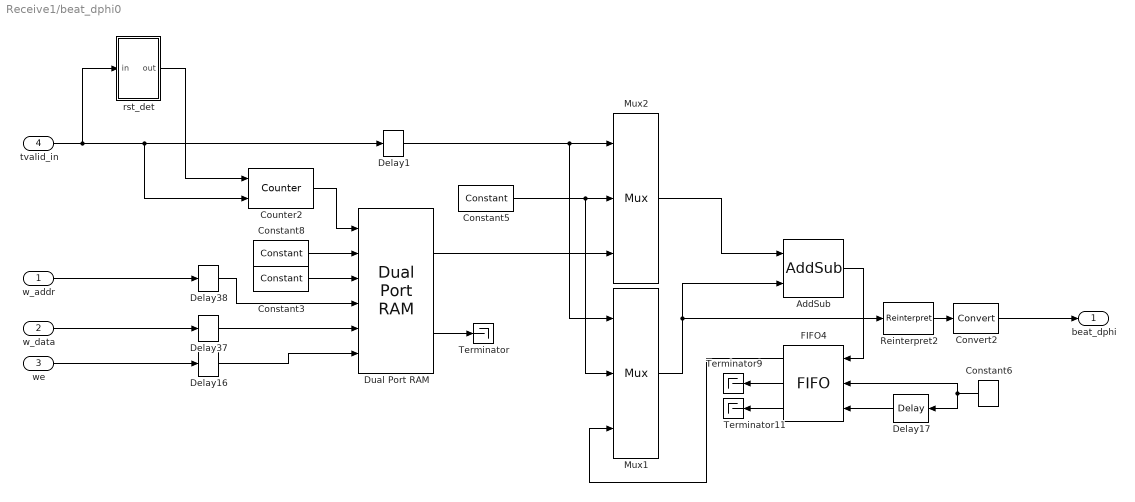
== system Receive1/beat_dphi0 ==
  w_addr : Inport
  w_data : Inport  Port=2
  we : Inport  Port=3
  tvalid_in : Inport  Port=4
  AddSub : xbsIndex_r4/AddSub  mode=Addition  use_carryin=off  use_carryout=off  en=off  latency=2  precision=User Defined  arith_type=Unsigned  n_bits=16  bin_pt=0  quantization=Truncate  overflow=Wrap  use_behavioral_HDL=off  hw_selection=Fabric  pipelined=off  dbl_ovrd=off  block_type=addsub
  Constant3 : xbsIndex_r4/Constant  const=0  gui_display_data_type=Boolean  arith_type=Boolean  n_bits=16  bin_pt=14  preci_type=Single  exp_width=8  frac_width=24  explicit_period=on  period=1  equ=P=C  opselect=C  inp2=PCIN>>17  opr=+  inp1=P  carry=CIN  dbl_ovrd=off  block_type=constant
  Constant5 : xbsIndex_r4/Constant  const=0  gui_display_data_type=Fixed-point  arith_type=Unsigned  n_bits=16  bin_pt=0  preci_type=Single  exp_width=8  frac_width=24  explicit_period=on  period=1  equ=P=C  opselect=C  inp2=PCIN>>17  opr=+  inp1=P  carry=CIN  dbl_ovrd=off  block_type=constant
  Constant6 : xbsIndex_r4/Constant  const=1  gui_display_data_type=Boolean  arith_type=Boolean  n_bits=16  bin_pt=14  preci_type=Single  exp_width=8  frac_width=24  explicit_period=on  period=1  equ=P=C  opselect=C  inp2=PCIN>>17  opr=+  inp1=P  carry=CIN  dbl_ovrd=off  block_type=constant
  Constant8 : xbsIndex_r4/Constant  const=0  gui_display_data_type=Fixed-point  arith_type=Unsigned  n_bits=16  bin_pt=0  preci_type=Single  exp_width=8  frac_width=24  explicit_period=on  period=1  equ=P=C  opselect=C  inp2=PCIN>>17  opr=+  inp1=P  carry=CIN  dbl_ovrd=off  block_type=constant
  Convert2 : xbsIndex_r4/Convert  gui_display_data_type=Fixed-point  arith_type="Signed  (2's comp)"  n_bits=18  bin_pt=15  float_type=Single  exp_bits=8  fraction_bits=24  quantization=Truncate  overflow=Wrap  en=off  latency=0  pipeline=off  dbl_ovrd=off  block_type=convert
  Counter2 : xbsIndex_r4/Counter  cnt_type=Free Running  cnt_to=Inf  operation=Up  start_count=0  cnt_by_val=1  arith_type=Unsigned  n_bits=9  bin_pt=0  load_pin=off  rst=on  en=on  explicit_period=on  period=1  use_behavioral_HDL=off  implementation=Fabric  dbl_ovrd=off  block_type=counter
  Delay{1,16,37..38} (4 alike) : xbsIndex_r4/Delay  rst=off  infoeditControl=Selection of Reset will increase slice count due to use of real FFs and instead of SRLs  en=off  latency=1  reg_retiming=off  dbl_ovrd=off  block_type=delay
  Delay17 : xbsIndex_r4/Delay  rst=off  infoeditControl=Selection of Reset will increase slice count due to use of real FFs and instead of SRLs  en=off  latency=n_overlapped_channel/parallel_factor-2-1-1  reg_retiming=off  dbl_ovrd=off  block_type=delay
  Dual Port RAM : xbsIndex_r4/Dual Port RAM  depth=n_overlapped_channel/parallel_factor  initVector=beat_dphi_uint16_0  distributed_mem=Block RAM  init_a=0  init_b=0  rst_a=off  rst_b=off  en_a=off  en_b=off  latency=1  write_mode_A=Read Before Write  write_mode_B=Read Before Write  optimize=Area  dbl_ovrd=off  simulation_type=fast_sim  block_type=dpram
  FIFO4 : xbsIndex_r4/FIFO  mem_type=Block RAM  performance_options=Standard_FIFO  embedded_registers=off  depth=1K  percent_nbits=1  rst=off  rst_latency=2  en=off  use_dcount=off  use_percent_full_port=off  use_almost_empty=off  almost_empty_thresh=2  use_almost_full=off  use_rd_rst_busy=off  use_wr_rst_busy=off  almost_full_thresh=14  explicit_period=off  dbl_ovrd=off  simulation_type=fast_sim  block_type=fifo
  Mux1 : xbsIndex_r4/Mux  inputs=2  en=off  latency=1  precision=User Defined  arith_type=Unsigned  n_bits=16  bin_pt=0  quantization=Truncate  overflow=Flag as error  dbl_ovrd=off  block_type=mux
  Mux2 : xbsIndex_r4/Mux  inputs=2  en=off  latency=1  precision=User Defined  arith_type=Unsigned  n_bits=16  bin_pt=0  quantization=Truncate  overflow=Flag as error  dbl_ovrd=off  block_type=mux
  Reinterpret2 : xbsIndex_r4/Reinterpret  force_arith_type=on  arith_type="Signed  (2's comp)"  force_bin_pt=on  bin_pt=15  block_type=reinterpret
  Terminator : Terminator
  Terminator11 : Terminator
  Terminator9 : Terminator
  rst_det : Subsystem
  beat_dphi : Outport
  wires:
  FIFO4/1 -> Mux1/3
  Reinterpret2/1 -> Convert2/1
  Delay17/1 -> FIFO4/3
  Delay38/1 -> Dual Port RAM/4
  Delay37/1 -> Dual Port RAM/5
  Delay16/1 -> Dual Port RAM/6
  Constant3/1 -> Dual Port RAM/3
  AddSub/1 -> FIFO4/1
  Constant6/1 -> FIFO4/2, Delay17/1
  FIFO4/3 -> Terminator11/1
  Constant8/1 -> Dual Port RAM/2
  FIFO4/2 -> Terminator9/1
  Dual Port RAM/2 -> Terminator/1
  Counter2/1 -> Dual Port RAM/1
  Constant5/1 -> Mux2/2, Mux1/2
  Mux2/1 -> AddSub/1
  w_data/1 -> Delay37/1
  Dual Port RAM/1 -> Mux2/3
  Convert2/1 -> beat_dphi/1
  w_addr/1 -> Delay38/1
  we/1 -> Delay16/1
  tvalid_in/1 -> rst_det/1(in), Delay1/1, Counter2/2
  rst_det/1(out) -> Counter2/1
  Delay1/1 -> Mux1/1, Mux2/1
  Mux1/1 -> Reinterpret2/1, AddSub/2

== system Receive1/beat_dphi1 ==
  w_addr : Inport
  w_data : Inport  Port=2
  we : Inport  Port=3
  tvalid_in : Inport  Port=4
  AddSub : xbsIndex_r4/AddSub  mode=Addition  use_carryin=off  use_carryout=off  en=off  latency=2  precision=User Defined  arith_type=Unsigned  n_bits=16  bin_pt=0  quantization=Truncate  overflow=Wrap  use_behavioral_HDL=off  hw_selection=Fabric  pipelined=off  dbl_ovrd=off  block_type=addsub
  Constant3 : xbsIndex_r4/Constant  const=0  gui_display_data_type=Boolean  arith_type=Boolean  n_bits=16  bin_pt=14  preci_type=Single  exp_width=8  frac_width=24  explicit_period=on  period=1  equ=P=C  opselect=C  inp2=PCIN>>17  opr=+  inp1=P  carry=CIN  dbl_ovrd=off  block_type=constant
  Constant5 : xbsIndex_r4/Constant  const=0  gui_display_data_type=Fixed-point  arith_type=Unsigned  n_bits=16  bin_pt=0  preci_type=Single  exp_width=8  frac_width=24  explicit_period=on  period=1  equ=P=C  opselect=C  inp2=PCIN>>17  opr=+  inp1=P  carry=CIN  dbl_ovrd=off  block_type=constant
  Constant6 : xbsIndex_r4/Constant  const=1  gui_display_data_type=Boolean  arith_type=Boolean  n_bits=16  bin_pt=14  preci_type=Single  exp_width=8  frac_width=24  explicit_period=on  period=1  equ=P=C  opselect=C  inp2=PCIN>>17  opr=+  inp1=P  carry=CIN  dbl_ovrd=off  block_type=constant
  Constant8 : xbsIndex_r4/Constant  const=0  gui_display_data_type=Fixed-point  arith_type=Unsigned  n_bits=16  bin_pt=0  preci_type=Single  exp_width=8  frac_width=24  explicit_period=on  period=1  equ=P=C  opselect=C  inp2=PCIN>>17  opr=+  inp1=P  carry=CIN  dbl_ovrd=off  block_type=constant
  Convert2 : xbsIndex_r4/Convert  gui_display_data_type=Fixed-point  arith_type="Signed  (2's comp)"  n_bits=18  bin_pt=15  float_type=Single  exp_bits=8  fraction_bits=24  quantization=Truncate  overflow=Wrap  en=off  latency=0  pipeline=off  dbl_ovrd=off  block_type=convert
  Counter2 : xbsIndex_r4/Counter  cnt_type=Free Running  cnt_to=Inf  operation=Up  start_count=0  cnt_by_val=1  arith_type=Unsigned  n_bits=9  bin_pt=0  load_pin=off  rst=on  en=on  explicit_period=on  period=1  use_behavioral_HDL=off  implementation=Fabric  dbl_ovrd=off  block_type=counter
  Delay{1,16,37..38} (4 alike) : xbsIndex_r4/Delay  rst=off  infoeditControl=Selection of Reset will increase slice count due to use of real FFs and instead of SRLs  en=off  latency=1  reg_retiming=off  dbl_ovrd=off  block_type=delay
  Delay17 : xbsIndex_r4/Delay  rst=off  infoeditControl=Selection of Reset will increase slice count due to use of real FFs and instead of SRLs  en=off  latency=n_overlapped_channel/parallel_factor-2-1-1  reg_retiming=off  dbl_ovrd=off  block_type=delay
  Dual Port RAM : xbsIndex_r4/Dual Port RAM  depth=n_overlapped_channel/parallel_factor  initVector=beat_dphi_uint16_1  distributed_mem=Block RAM  init_a=0  init_b=0  rst_a=off  rst_b=off  en_a=off  en_b=off  latency=1  write_mode_A=Read Before Write  write_mode_B=Read Before Write  optimize=Area  dbl_ovrd=off  simulation_type=fast_sim  block_type=dpram
  FIFO4 : xbsIndex_r4/FIFO  mem_type=Block RAM  performance_options=Standard_FIFO  embedded_registers=off  depth=1K  percent_nbits=1  rst=off  rst_latency=2  en=off  use_dcount=off  use_percent_full_port=off  use_almost_empty=off  almost_empty_thresh=2  use_almost_full=off  use_rd_rst_busy=off  use_wr_rst_busy=off  almost_full_thresh=14  explicit_period=off  dbl_ovrd=off  simulation_type=fast_sim  block_type=fifo
  Mux1 : xbsIndex_r4/Mux  inputs=2  en=off  latency=1  precision=User Defined  arith_type=Unsigned  n_bits=16  bin_pt=0  quantization=Truncate  overflow=Flag as error  dbl_ovrd=off  block_type=mux
  Mux2 : xbsIndex_r4/Mux  inputs=2  en=off  latency=1  precision=User Defined  arith_type=Unsigned  n_bits=16  bin_pt=0  quantization=Truncate  overflow=Flag as error  dbl_ovrd=off  block_type=mux
  Reinterpret2 : xbsIndex_r4/Reinterpret  force_arith_type=on  arith_type="Signed  (2's comp)"  force_bin_pt=on  bin_pt=15  block_type=reinterpret
  Terminator : Terminator
  Terminator11 : Terminator
  Terminator9 : Terminator
  rst_det : Subsystem
  beat_dphi : Outport
  wires:
  FIFO4/1 -> Mux1/3
  Reinterpret2/1 -> Convert2/1
  Delay17/1 -> FIFO4/3
  Delay38/1 -> Dual Port RAM/4
  Delay37/1 -> Dual Port RAM/5
  Delay16/1 -> Dual Port RAM/6
  Constant3/1 -> Dual Port RAM/3
  AddSub/1 -> FIFO4/1
  Constant6/1 -> FIFO4/2, Delay17/1
  FIFO4/3 -> Terminator11/1
  Constant8/1 -> Dual Port RAM/2
  FIFO4/2 -> Terminator9/1
  Dual Port RAM/2 -> Terminator/1
  Counter2/1 -> Dual Port RAM/1
  Constant5/1 -> Mux2/2, Mux1/2
  Mux2/1 -> AddSub/1
  w_data/1 -> Delay37/1
  Dual Port RAM/1 -> Mux2/3
  Convert2/1 -> beat_dphi/1
  w_addr/1 -> Delay38/1
  we/1 -> Delay16/1
  tvalid_in/1 -> rst_det/1(in), Delay1/1, Counter2/2
  rst_det/1(out) -> Counter2/1
  Delay1/1 -> Mux1/1, Mux2/1
  Mux1/1 -> Reinterpret2/1, AddSub/2
